simulink model "Serial_example"  (R2022a)
settings: Solver=FixedStepAuto  StartTime=0.0  StopTime=10.0  FixedStep=1e-3  RelTol=1e-3  EnableMultiTasking=on
libraries: frdmk64flib x5, etargetslib x2
settings Model: ExtModeTrigDuration=5  Creator=haotianxue  LastModifiedBy=liaml
settings OptimizationCC: EnhancedBackFolding=on  PassReuseOutputArgsAs=Individual arguments  ZeroExternalMemoryAtStartup=off  ZeroInternalMemoryAtStartup=off  MaxStackSize=64  OptimizeBlockOrder=speed  DifferentSizesBufferReuse=on  OptimizationCustomize=off  EfficientTunableParamExpr=on
settings DebuggingCC: ParameterTunabilityLossMsg=error  UnconnectedInputMsg=warning  UnconnectedOutputMsg=warning  UnconnectedLineMsg=warning
settings HardwareCC: ProdBitPerPointer=32  ProdBitPerSizeT=32  ProdBitPerPtrDiffT=32  ProdLargestAtomicInteger=Long  ProdLargestAtomicFloat=Double  ProdWordSize=32  ProdHWDeviceType=ARM Compatible->ARM Cortex
settings SFSimCC: MATLABDynamicMemAlloc=off
settings RTWCC: SystemTargetFile=ert.tlc  HardwareBoard=NXP FRDM-K64F  TLCOptions="-aInlineSetEventsForThisBaseRateFcn=TLC_FALSE -aSuppressMultiTaskScheduler=TLC_FALSE  -aRateBasedStepFcn=0"  TemplateMakefile=ert_default_tmf  Toolchain=GNU Tools for ARM Embedded Processors  DLArmComputeVersion=19.05
settings CodeAppCC: ForceParamTrailComments=on  IgnoreCustomStorageClasses=off  OperatorAnnotations=on  SimulinkDataObjDesc=on  SFDataObjDesc=on  InsertBlockDesc=on
settings ERTTargetCC: ExtModeTransport=4  ExtModeMexFile=sendToCommService

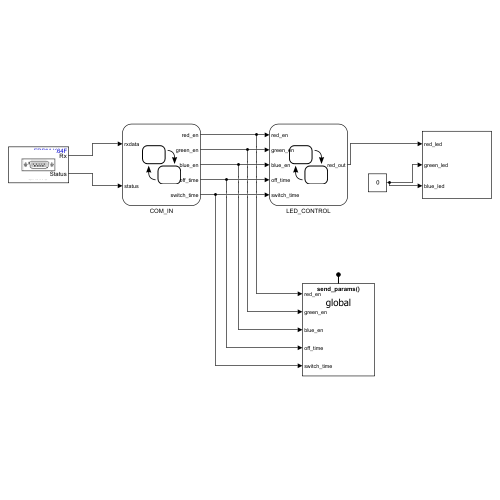
[thumbnail: Simulink's stored preview of the top-level diagram]
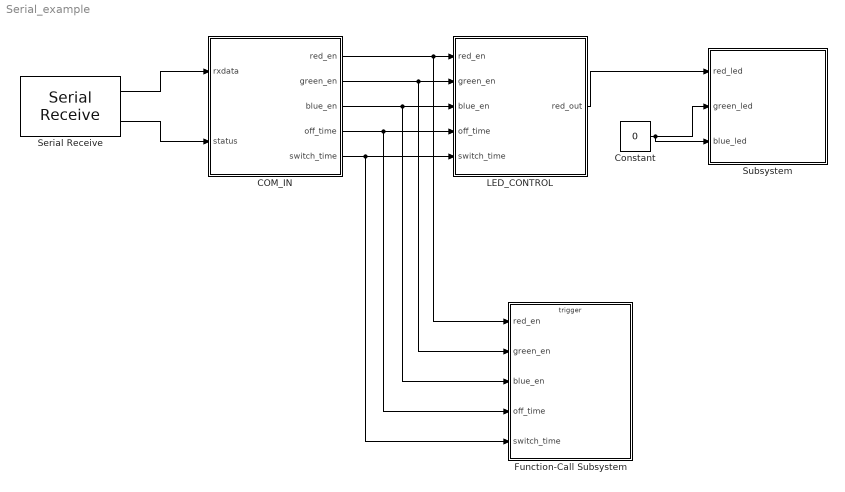
== system Serial_example ==
  COM_IN : Stateflow chart  TreatAsAtomicUnit=on
  Constant : Constant  Value=0
  Function-Call Subsystem : Subsystem  TreatAsAtomicUnit=on
  LED_CONTROL : Stateflow chart  TreatAsAtomicUnit=on
  Serial Receive : frdmk64flib/Serial Receive  SCIModule=0  Baudrate=uint32(9600)  Parity=None  StopBits=1  HardwareFlowControl=None  ByteOrder=LittleEndian  DataType=uint8  DataLength=11  BlockingMode=off  OutputStatus=on  SampleTime=-1
  Subsystem : Subsystem
  wires:
  Serial Receive/1 -> COM_IN/1(rxdata)
  Serial Receive/2 -> COM_IN/2(status)
  LED_CONTROL/1(red_out) -> Subsystem/1(red_led)
  COM_IN/5(switch_time) -> Function-Call Subsystem/5(switch_time), LED_CONTROL/5(switch_time)
  COM_IN/1(red_en) -> Function-Call Subsystem/1(red_en), LED_CONTROL/1(red_en)
  COM_IN/4(off_time) -> Function-Call Subsystem/4(off_time), LED_CONTROL/4(off_time)
  COM_IN/2(green_en) -> Function-Call Subsystem/2(green_en), LED_CONTROL/2(green_en)
  COM_IN/3(blue_en) -> Function-Call Subsystem/3(blue_en), LED_CONTROL/3(blue_en)
  Constant/1 -> Subsystem/3(blue_led), Subsystem/2(green_led)

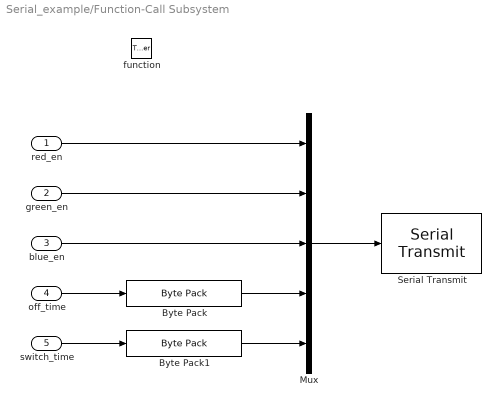
== system Serial_example/Function-Call Subsystem ==
  red_en : Inport
  green_en : Inport  Port=2
  blue_en : Inport  Port=3
  off_time : Inport  Port=4
  switch_time : Inport  Port=5
  function : TriggerPort  TriggerType=function-call  IsSimulinkFunction=on  FunctionName=send_params  VariantControl=(inherit)
  Byte Pack : etargetslib/Byte Pack  datatypes={'single'}  byteAlign=1
  Byte Pack1 : etargetslib/Byte Pack  datatypes={'uint16'}  byteAlign=1
  Mux : Mux  Inputs=5
  Serial Transmit : frdmk64flib/Serial Transmit  SCIModule=0  Baudrate=uint32(9600)  Parity=None  StopBits=1  HardwareFlowControl=None  ByteOrder=LittleEndian  BlockingMode=on  OutputStatus=off
  wires:
  off_time/1 -> Byte Pack/1
  switch_time/1 -> Byte Pack1/1
  Mux/1 -> Serial Transmit/1
  red_en/1 -> Mux/1
  green_en/1 -> Mux/2
  blue_en/1 -> Mux/3
  Byte Pack/1 -> Mux/4
  Byte Pack1/1 -> Mux/5

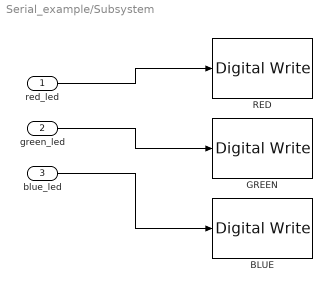
== system Serial_example/Subsystem ==
  red_led : Inport
  green_led : Inport  Port=2
  blue_led : Inport  Port=3
  BLUE : frdmk64flib/Digital Write  Whichpin=BLUE_LED
  GREEN : frdmk64flib/Digital Write  Whichpin=GREEN_LED
  RED : frdmk64flib/Digital Write  Whichpin=RED_LED
  wires:
  blue_led/1 -> BLUE/1
  red_led/1 -> RED/1
  green_led/1 -> GREEN/1

== stateflow chart Serial_example/LED_CONTROL ==
  state RED_OFF
    entry:
    red_out=false;
  state OFF
    entry:
    red_out=false;
  state RED_ON
    entry:
    red_out=true;
  RED_OFF -> (junction 14)
  (junction 14) -> RED_OFF [order 2] : [red_en==0]
  (default) -> OFF
  OFF -> (junction 14) : after(off_time,sec)
  (junction 14) -> RED_ON [order 1] : [red_en==1]
  RED_ON -> (junction 14)
  data: red_en input uint8; green_en input uint8; blue_en input uint8; off_time input single; red_out output boolean; switch_time input uint16

== stateflow chart Serial_example/COM_IN ==
  state SET_PARAM
    entry:
    red_en = rxdata(3);
    green_en =  rxdata(4);
    blue_en = rxdata(5);
    off_time = typecast(rxdata(6:9), 'sinlge');
    switch_time = typecast(rxdata(10:11), 'uint16');
  state INITIAL
    entry:
    red_en = 0;
    green_en = 0;
    blue_en = 0;
    off_time = 0.5;
    switch_time = 200;
  state STANDBY
  state ECHO_PARAM
    entry:
    send_params();
  SET_PARAM -> STANDBY
  (junction 15) -> SET_PARAM [order 1] : [rxdata(2)==hex2dec('55')]
  (default) -> INITIAL
  (junction 14) -> STANDBY [order 2]
  INITIAL -> STANDBY
  STANDBY -> (junction 14) : [status==0]
  (junction 14) -> (junction 15) [order 1] : [rxdata(1)==hex2dec('16')]
  (junction 15) -> ECHO_PARAM [order 2] : [rxdata(2)==hex2dec('22')]
  ECHO_PARAM -> STANDBY
  data: rxdata input uint8; status input uint8; red_en output uint8; green_en output uint8; blue_en output uint8; off_time output single; switch_time output uint16
